simulink model "Virtual_Exhaust_Aftertreatment_Controller_PRT"  (R2016b)
settings: Solver=FixedStepAuto  StartTime=0.0  StopTime=inf  FixedStep=VirtExhATCtrlr.tiSimnTiStep_C  RelTol=1e-3  SampleTimeConstraint=STIndependent  EnableMultiTasking=on
undefined symbols (not defined in the file or in its folder): CAL, SOUIT, T3LIMCL_COEOM_MSK_SY, T3LimCL_stMskEOM1_C, T3LimCL_stMskEOM2_C, T3LimCL_stMskEOM3_C, VirtExhATCtrlr_numHrznSize_CA
libraries: simulink x4
(part 4 of 5)

== system Virtual_Exhaust_Aftertreatment_Controller_PRT/UCatCtrl/Urea_Dosing_Control/Load Governor/Saturation Dynamic ==
  up : Inport
  u : Inport  Port=2
  lo : Inport  Port=3
  Data Type Duplicate : DataTypeDuplicate  DisableCoverage=on
  Data Type Propagation : S-Function  FunctionName=sfix_dtprop  Parameters=14,PropDataTypeMode,(getdatatypespecs(PropDataType,PropScaling,DblOver,0, 0, PropDataTypeMode, PropScalingMode)),IfRefDouble,IfRefSingle,IsSigned,NumBitsBase,NumBitsMult,NumBitsAdd,(sort(reshape(round(NumBitsAllowFinal), prod(size(NumBitsAllowFinal)),1))),PropScalingMode,ValuesUsedBestPrec,SlopeBase,SlopeMult,SlopeAdd,BiasBase,BiasMult,BiasAdd,DblOver  SFunctionDeploymentMode=off  EnableBusSupport=off  mask(Data Type Propagation){PropDataTypeMode=Inherit via propagation rule, PropDataType=fixdt(1, 16), IfRefDouble=double, IfRefSingle=single, IsSigned=IsSigned1, NumBitsBase=NumBits1, NumBitsMult=1, NumBitsAdd=0, NumBitsAllowFinal=1:128, PropScalingMode=Inherit via propagation rule, PropScaling=2^-10, ValuesUsedBestPrec=[5 -7], SlopeBase=Slope1, SlopeMult=1, SlopeAdd=0, BiasBase=Bias1, BiasMult=1, BiasAdd=0}
      mask prompts: PropDataTypeMode "Simulink:masks:x1PropagatedDataType_MP"; PropDataType "Simulink:masks:x11PropagatedDataTypeegFixdt116Fixdtsingle_MP"; IfRefDouble "Simulink:masks:x11IfAnyReferenceInputIsDoubleOutputIs_MP"; IfRefSingle "Simulink:masks:x12IfAnyReferenceInputIsSingleOutputIs_MP"; IsSigned "Simulink:masks:x13IsSigned_MP"; NumBitsBase "Simulink:masks:x141NumberofBitsBase_MP"; NumBitsMult "Simulink:masks:x142NumberofBitsMultiplicativeAdjustment_MP"; NumBitsAdd "Simulink:masks:x143NumberofBitsAdditiveAdjustment_MP"; NumBitsAllowFinal "Simulink:masks:x144NumberofBitsAllowableFinalValues_MP"; PropScalingMode "Simulink:masks:x2PropagatedScaling_MP"; PropScaling "Simulink:masks:x21PropagatedScalingSlopeEg29OrSlopeBiasEg1253_MP"; ValuesUsedBestPrec "Simulink:masks:x21ValuesUsedToDetermineBestPrecisionScaling_MP"; SlopeBase "Simulink:masks:x211SlopeBase_MP"; SlopeMult "Simulink:masks:x212SlopeMultiplicativeAdjustment_MP"; SlopeAdd "Simulink:masks:x213SlopeAdditiveAdjustment_MP"; BiasBase "Simulink:masks:x221BiasBase_MP"; BiasMult "Simulink:masks:x222BiasMultiplicativeAdjustment_MP"; BiasAdd "Simulink:masks:x223BiasAdditiveAdjustment_MP"
      mask help: Simulink:masks:DataTypePropagation_MD
      mask init:
      | DblOver = 0;
      mask TypeOptions PropDataTypeMode: Simulink:masks:SpecifyViaDialog | Simulink:masks:InheritViaPropagationRule
      mask Callback PropDataTypeMode: fixptdialog(gcbh)
      mask Callback PropDataType: fixptdialog(gcbh)
      mask TypeOptions IfRefDouble: Simulink:masks:double | Simulink:masks:single
      mask TypeOptions IfRefSingle: Simulink:masks:double | Simulink:masks:single
      mask TypeOptions IsSigned: Simulink:masks:IsSigned1 | Simulink:masks:IsSigned2 | Simulink:masks:IsSigned1OrIsSigned2 | Simulink:masks:TRUE | Simulink:masks:FALSE
      mask TypeOptions NumBitsBase: NumBits1 | NumBits2 | max([NumBits1 NumBits2]) | min([NumBits1 NumBits2]) | NumBits1+NumBits2
      mask TypeOptions PropScalingMode: Simulink:masks:SpecifyViaDialog | Simulink:masks:InheritViaPropagationRule | Simulink:masks:ObtainViaBestPrecision
      mask Callback PropScalingMode: fixptdialog(gcbh)
      mask TypeOptions SlopeBase: Slope1 | Slope2 | max([Slope1 Slope2]) | min([Slope1 Slope2]) | Slope1*Slope2 | Slope1/Slope2 | PosRange1 | PosRange2 | max([PosRange1 PosRange2]) | min([PosRange1 PosRange2]) | PosRange1*PosRange2 | PosRange1/PosRange2
      mask TypeOptions BiasBase: Bias1 | Bias2 | max([Bias1 Bias2]) | min([Bias1 Bias2]) | Bias1*Bias2 | Bias1/Bias2 | Bias1+Bias2 | Bias1-Bias2
      mask Display:
      | port_label('Input',1,'Ref1');
      | port_label('Input',2,'Ref2');
      | port_label('Input',3,'Prop');
  LowerRelop1 : RelationalOperator  DisableCoverage=on  Operator=>  OutDataTypeStr=boolean  RndMeth=Nearest
  Switch : Switch  Criteria=u2 ~= 0  OutDataTypeStr=Inherit: Inherit via back propagation  ZeroCross=off
  Switch2 : Switch  Criteria=u2 ~= 0  OutMin=OutMin  OutMax=OutMax  OutDataTypeStr=Inherit: Inherit via back propagation  ZeroCross=off
  UpperRelop : RelationalOperator  DisableCoverage=on  Operator=<  OutDataTypeStr=boolean  RndMeth=Nearest
  y : Outport  OutMin=OutMin  OutMax=OutMax
  wires:
  up/1 -> Switch2/1, LowerRelop1/2
  u/1 -> Data Type Propagation/2, Data Type Propagation/1, LowerRelop1/1, Switch/3, UpperRelop/1
  lo/1 -> Switch/1, UpperRelop/2
  Switch/1 -> Data Type Duplicate/2, Switch2/3, Data Type Propagation/3
  Switch2/1 -> Data Type Duplicate/1, y/1
  LowerRelop1/1 -> Switch2/2
  UpperRelop/1 -> Switch/2

== system Virtual_Exhaust_Aftertreatment_Controller_PRT/UCatCtrl/SCR_Prediction/Main/Aging Prediction/estAging ==
  ATS_tAvrg : Inport
  ATS_GlbDa_ITotDst : Inport  Port=2
  Constant1 : Constant  Value=CAL.SCALAR.SCRMod_facSCRAgeSca_C  OutDataTypeStr=Inherit: Inherit via back propagation  SampleTime=-1
  Constant10 : Constant  Value=CAL.SCALAR.SCRMod_facSCRAgeTempSca_C  OutDataTypeStr=Inherit: Inherit via back propagation  SampleTime=-1
  Constant2 : Constant  Value=32767  SampleTime=-1
  MinMax : MinMax  Inputs=2
  MinMax1 : MinMax  Inputs=2
  Product : Product
  Product1 : Product
  SCRMod_facEffSCRAge_MAP : Lookup_n-D  BreakpointsForDimension1=CAL.TABLE.SCRMod_facEffSCRAge_MAP.Y  BreakpointsForDimension2=CAL.TABLE.SCRMod_facEffSCRAge_MAP.X  Table=CAL.TABLE.SCRMod_facEffSCRAge_MAP.Z  ExtrapMethod=Clip  UseLastTableValue=on  RndMeth=Simplest  InputSameDT=on
  SCRMod_facTempSCRAge_CUR : Lookup_n-D  NumberOfTableDimensions=1  BreakpointsForDimension1=CAL.TABLE.SCRMod_facTempSCRAge_MAP.X  BreakpointsForDimension2=CAL.TABLE.SCRMod_facEffSCRAge_MAP.X  Table=CAL.TABLE.SCRMod_facTempSCRAge_MAP.Y  ExtrapMethod=Clip  UseLastTableValue=on  RndMeth=Simplest  InputSameDT=on
  ATS_facEstEfcUCatAge : Outport
  wires:
  ATS_tAvrg/1 -> SCRMod_facTempSCRAge_CUR/1
  SCRMod_facTempSCRAge_CUR/1 -> Product1/1
  Constant10/1 -> Product1/2
  Product1/1 -> MinMax/1
  Constant2/1 -> MinMax1/1, MinMax/2
  Product/1 -> MinMax1/2
  MinMax/1 -> SCRMod_facEffSCRAge_MAP/1
  MinMax1/1 -> SCRMod_facEffSCRAge_MAP/2
  SCRMod_facEffSCRAge_MAP/1 -> ATS_facEstEfcUCatAge/1
  ATS_GlbDa_ITotDst/1 -> Product/1
  Constant1/1 -> Product/2

== system Virtual_Exhaust_Aftertreatment_Controller_PRT/UCatCtrl/SCR_Prediction/Main/UCat Efficiency Prediction/SubSystem_10 ==
  In1 : Inport
  In2 : Inport  Port=2
  In3 : Inport  Port=3
  In4 : Inport  Port=4
  Interpolation Using Prelookup : Interpolation_n-D  Table=table  ExtrapMethod=Clip  ValidIndexMayReachLast=on
  Out1 : Outport
  wires:
  Interpolation Using Prelookup/1 -> Out1/1
  In1/1 -> Interpolation Using Prelookup/1
  In2/1 -> Interpolation Using Prelookup/2
  In3/1 -> Interpolation Using Prelookup/3
  In4/1 -> Interpolation Using Prelookup/4

== system Virtual_Exhaust_Aftertreatment_Controller_PRT/UCatCtrl/SCR_Prediction/Main/UCat Efficiency Prediction/SubSystem_11 ==
  In1 : Inport
  In2 : Inport  Port=2
  In3 : Inport  Port=3
  In4 : Inport  Port=4
  Interpolation Using Prelookup : Interpolation_n-D  Table=table  ExtrapMethod=Clip  ValidIndexMayReachLast=on
  Out1 : Outport
  wires:
  In4/1 -> Interpolation Using Prelookup/4
  In3/1 -> Interpolation Using Prelookup/3
  In2/1 -> Interpolation Using Prelookup/2
  In1/1 -> Interpolation Using Prelookup/1
  Interpolation Using Prelookup/1 -> Out1/1

== system Virtual_Exhaust_Aftertreatment_Controller_PRT/UCatCtrl/SCR_Prediction/Main/UCat Efficiency Prediction/SubSystem_12 ==
  In1 : Inport
  In2 : Inport  Port=2
  In3 : Inport  Port=3
  In4 : Inport  Port=4
  Interpolation Using Prelookup : Interpolation_n-D  Table=table  ExtrapMethod=Clip  ValidIndexMayReachLast=on
  Out1 : Outport
  wires:
  In4/1 -> Interpolation Using Prelookup/4
  In3/1 -> Interpolation Using Prelookup/3
  In2/1 -> Interpolation Using Prelookup/2
  In1/1 -> Interpolation Using Prelookup/1
  Interpolation Using Prelookup/1 -> Out1/1

== system Virtual_Exhaust_Aftertreatment_Controller_PRT/UCatCtrl/SCR_Prediction/Main/UCat Efficiency Prediction/SubSystem_3 ==
  In1 : Inport
  In2 : Inport  Port=2
  In3 : Inport  Port=3
  In4 : Inport  Port=4
  Interpolation Using Prelookup : Interpolation_n-D  Table=table  ExtrapMethod=Clip  ValidIndexMayReachLast=on
  Out1 : Outport
  wires:
  Interpolation Using Prelookup/1 -> Out1/1
  In1/1 -> Interpolation Using Prelookup/1
  In2/1 -> Interpolation Using Prelookup/2
  In3/1 -> Interpolation Using Prelookup/3
  In4/1 -> Interpolation Using Prelookup/4

== system Virtual_Exhaust_Aftertreatment_Controller_PRT/UCatCtrl/SCR_Prediction/Main/UCat Efficiency Prediction/SubSystem_4 ==
  In1 : Inport
  In2 : Inport  Port=2
  In3 : Inport  Port=3
  In4 : Inport  Port=4
  Interpolation Using Prelookup : Interpolation_n-D  Table=table  ExtrapMethod=Clip  ValidIndexMayReachLast=on
  Out1 : Outport
  wires:
  In4/1 -> Interpolation Using Prelookup/4
  In3/1 -> Interpolation Using Prelookup/3
  In2/1 -> Interpolation Using Prelookup/2
  In1/1 -> Interpolation Using Prelookup/1
  Interpolation Using Prelookup/1 -> Out1/1

== system Virtual_Exhaust_Aftertreatment_Controller_PRT/UCatCtrl/SCR_Prediction/Main/UCat Efficiency Prediction/SubSystem_5 ==
  In1 : Inport
  In2 : Inport  Port=2
  In3 : Inport  Port=3
  In4 : Inport  Port=4
  Interpolation Using Prelookup : Interpolation_n-D  Table=table  ExtrapMethod=Clip  ValidIndexMayReachLast=on
  Out1 : Outport
  wires:
  Interpolation Using Prelookup/1 -> Out1/1
  In1/1 -> Interpolation Using Prelookup/1
  In2/1 -> Interpolation Using Prelookup/2
  In3/1 -> Interpolation Using Prelookup/3
  In4/1 -> Interpolation Using Prelookup/4

== system Virtual_Exhaust_Aftertreatment_Controller_PRT/UCatCtrl/SCR_Prediction/Main/UCat Efficiency Prediction/SubSystem_6 ==
  In1 : Inport
  In2 : Inport  Port=2
  In3 : Inport  Port=3
  In4 : Inport  Port=4
  Interpolation Using Prelookup : Interpolation_n-D  Table=table  ExtrapMethod=Clip  ValidIndexMayReachLast=on
  Out1 : Outport
  wires:
  In4/1 -> Interpolation Using Prelookup/4
  In3/1 -> Interpolation Using Prelookup/3
  In2/1 -> Interpolation Using Prelookup/2
  In1/1 -> Interpolation Using Prelookup/1
  Interpolation Using Prelookup/1 -> Out1/1

== system Virtual_Exhaust_Aftertreatment_Controller_PRT/UCatCtrl/SCR_Prediction/Main/UCat Efficiency Prediction/SubSystem_7 ==
  In1 : Inport
  In2 : Inport  Port=2
  In3 : Inport  Port=3
  In4 : Inport  Port=4
  Interpolation Using Prelookup : Interpolation_n-D  Table=table  ExtrapMethod=Clip  ValidIndexMayReachLast=on
  Out1 : Outport
  wires:
  Interpolation Using Prelookup/1 -> Out1/1
  In1/1 -> Interpolation Using Prelookup/1
  In2/1 -> Interpolation Using Prelookup/2
  In3/1 -> Interpolation Using Prelookup/3
  In4/1 -> Interpolation Using Prelookup/4

== system Virtual_Exhaust_Aftertreatment_Controller_PRT/UCatCtrl/SCR_Prediction/Main/UCat Efficiency Prediction/SubSystem_8 ==
  In1 : Inport
  In2 : Inport  Port=2
  In3 : Inport  Port=3
  In4 : Inport  Port=4
  Interpolation Using Prelookup : Interpolation_n-D  Table=table  ExtrapMethod=Clip  ValidIndexMayReachLast=on
  Out1 : Outport
  wires:
  Interpolation Using Prelookup/1 -> Out1/1
  In1/1 -> Interpolation Using Prelookup/1
  In2/1 -> Interpolation Using Prelookup/2
  In3/1 -> Interpolation Using Prelookup/3
  In4/1 -> Interpolation Using Prelookup/4

== system Virtual_Exhaust_Aftertreatment_Controller_PRT/UCatCtrl/SCR_Prediction/Main/UCat Efficiency Prediction/SubSystem_9 ==
  In1 : Inport
  In2 : Inport  Port=2
  In3 : Inport  Port=3
  In4 : Inport  Port=4
  Interpolation Using Prelookup : Interpolation_n-D  Table=table  ExtrapMethod=Clip  ValidIndexMayReachLast=on
  Out1 : Outport
  wires:
  In4/1 -> Interpolation Using Prelookup/4
  In3/1 -> Interpolation Using Prelookup/3
  In2/1 -> Interpolation Using Prelookup/2
  In1/1 -> Interpolation Using Prelookup/1
  Interpolation Using Prelookup/1 -> Out1/1

== system Virtual_Exhaust_Aftertreatment_Controller_PRT/UCatCtrl/SCR_Prediction/Main/UCat NH3 Load Prediction/Discrete Integrator ==
  X : Inport
  Ki : Inport  Port=2
  Reset : Inport  Port=3
  Y0_YReset : Inport  Port=4
  Min : Inport  Port=5
  Max : Inport  Port=6
  dT : Inport  Port=7
  Add1 : Sum
  Add2 : Sum
  AntiWindUp : Subsystem
  Constant2 : Constant  Value=0  SampleTime=-1
  Constant3 : Constant  Value=0  SampleTime=-1
  Kp = 0 : Constant  SampleTime=-1
  Product1 : Product  RndMeth=Zero
  Product2 : Product  RndMeth=Zero
  Product3 : Product  RndMeth=Zero
  Saturation : Subsystem
  Switch1 : Switch  Criteria=u2 ~= 0
  Switch2 : Switch  Criteria=u2 ~= 0
  Switch3 : Switch  Criteria=u2 ~= 0
  Unit Delay External IC : Subsystem  mask(Unit Delay External Initial Condition){tsamp=-1}
      mask prompts: tsamp "Simulink:masks:SampleTime_MP"
      mask help: Simulink:masks:UnitDelayExternalInitialCondition_MD
      mask Display: dpoly(1,[1 0],'z')
  Unit Delay External IC1 : Subsystem  mask(Unit Delay External Initial Condition){tsamp=-1}
      mask prompts: tsamp "Simulink:masks:SampleTime_MP"
      mask help: Simulink:masks:UnitDelayExternalInitialCondition_MD
      mask Display: dpoly(1,[1 0],'z')
  Y : Outport
  wires:
  Unit Delay External IC1/1(y) -> Y/1
  X/1 -> Product2/1, Product1/1
  Kp = 0/1 -> Product1/2
  Ki/1 -> Product2/2
  Product2/1 -> Product3/1
  dT/1 -> Product3/2
  Product3/1 -> AntiWindUp/1(PreInteg), Switch1/3
  Unit Delay External IC/1(y) -> Add1/2
  Max/1 -> Saturation/1(Max)
  Min/1 -> Saturation/3(Min)
  Switch1/1 -> Add1/1
  Constant2/1 -> Switch1/1
  AntiWindUp/1(Clamp) -> Switch1/2
  Saturation/2(Sat) -> AntiWindUp/2(Sat)
  Add1/1 -> Switch2/3
  Reset/1 -> Switch2/2, Switch3/2
  Y0_YReset/1 -> Switch2/1, Unit Delay External IC/2(IC), Unit Delay External IC1/2(IC)
  Product1/1 -> Switch3/3
  Constant3/1 -> Switch3/1
  Saturation/1(Y) -> Unit Delay External IC/1(u), Add2/2
  Switch3/1 -> Add2/1
  Add2/1 -> Unit Delay External IC1/1(u)
  Switch2/1 -> Saturation/2(X)

== system Virtual_Exhaust_Aftertreatment_Controller_PRT/UCatCtrl/SCR_Prediction/Main/UCat NH3 Load Prediction/GOTO_ATS_mflNH3OxiUCatUs_mgps ==
  InXX : Inport
  GainXX : Subsystem
  tag scope: ATS_mflNH3OxiUCatUs_mgps=global
  wires:
  GainXX/1(Out) -> [ATS_mflNH3OxiUCatUs_mgps]  "ATS_mflNH3OxiUCatUs_mgps"
  InXX/1 -> GainXX/1(In)

== system Virtual_Exhaust_Aftertreatment_Controller_PRT/UCatCtrl/SCR_Prediction/Main/UCat NH3 Load Prediction/NH3 Oxidation ==
  ATS_tEstUCatAvrg : Inport
  ATS_mflEG : Inport  Port=2
  ATS_mflNH3MetAdapDes_mgps : Inport  Port=3
  ATS_facEffUCatAge : Inport  Port=4
  ATS_mEstNH3LdUCat : Inport  Port=5
  NH3 Oxidation : Subsystem
  mg/s to ppm : Subsystem
  ATS_mflNH3OxiUCatUs_mgps : Outport
  wires:
  ATS_tEstUCatAvrg/1 -> NH3 Oxidation/2(ATS_tEstUCatAvrg)
  ATS_mEstNH3LdUCat/1 -> NH3 Oxidation/1(ATS_mEstNH3LdUCat)
  ATS_mflEG/1 -> NH3 Oxidation/4("ATS_mflEG "), mg/s to ppm/2(ATS_mflEG)
  ATS_mflNH3MetAdapDes_mgps/1 -> mg/s to ppm/1(ATS_mflNH3MetAdapDes_mgps)
  mg/s to ppm/1(ATS_rNH3Curr_ppm) -> NH3 Oxidation/3(ATS_rNH3Curr_ppm)
  ATS_facEffUCatAge/1 -> NH3 Oxidation/5(ATS_facEffUCatAge)
  NH3 Oxidation/1(ATS_mflNH3OxiUCatUs_mgps) -> ATS_mflNH3OxiUCatUs_mgps/1

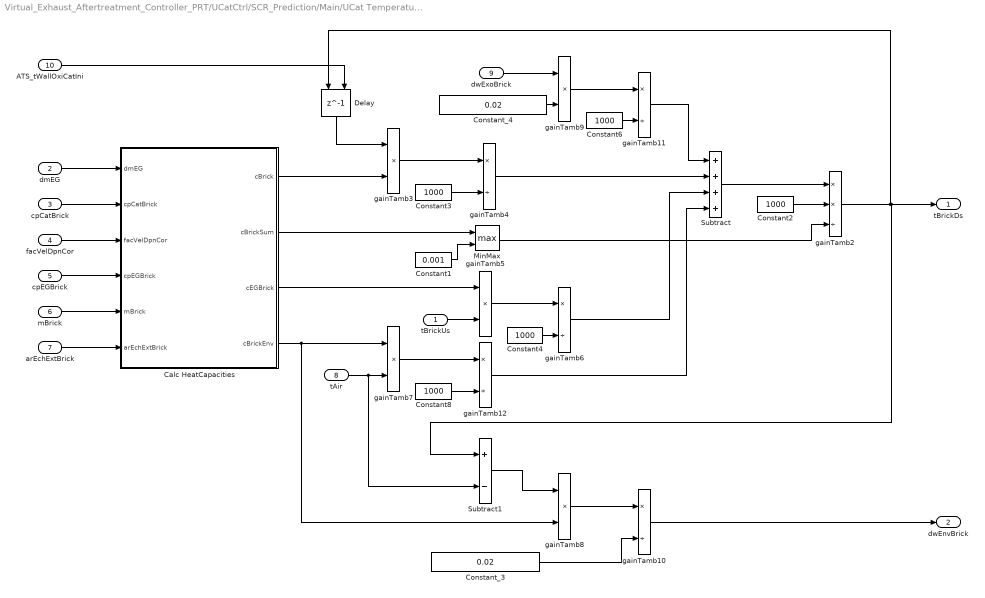
== system Virtual_Exhaust_Aftertreatment_Controller_PRT/UCatCtrl/SCR_Prediction/Main/UCat Temperature Prediction/DOC Temperature Estimation 1 ==
  tBrickUs : Inport
  dmEG : Inport  Port=2
  cpCatBrick : Inport  Port=3
  facVelDpnCor : Inport  Port=4
  cpEGBrick : Inport  Port=5
  mBrick : Inport  Port=6
  arEchExtBrick : Inport  Port=7
  tAir : Inport  Port=8
  dwExoBrick : Inport  Port=9
  ATS_tWallOxiCatIni : Inport  Port=10
  Calc HeatCapacities : Subsystem  TreatAsAtomicUnit=on
  Constant1 : Constant  Value=0.001  SampleTime=-1
  Constant{2..4,6,8} (5 alike) : Constant  Value=1000  SampleTime=-1
  Constant_3 : Constant  Value=0.02  SampleTime=-1
  Constant_4 : Constant  Value=0.02  SampleTime=-1
  Delay : Delay  DelayLength=1  InitialConditionSource=Input port  InitialCondition=0
      settings: InputPortMap=u0,p4
  MinMax : MinMax  Function=max  Inputs=2
  Subtract : Sum  Inputs=++++
  Subtract1 : Sum  Inputs=+-
  gainTamb{4,6,10..12} (5 alike) : Product  Inputs=*/  SaturateOnIntegerOverflow=on  InputSameDT=on  OutDataTypeStr=Inherit: Same as first input
  gainTamb2 : Product  Inputs=**/  SaturateOnIntegerOverflow=on  InputSameDT=on  OutDataTypeStr=Inherit: Same as first input
  gainTamb{3,5,7..9} (5 alike) : Product  Inputs=**  SaturateOnIntegerOverflow=on  InputSameDT=on  OutDataTypeStr=Inherit: Same as first input
  tBrickDs : Outport
  dwEnvBrick : Outport  Port=2
  wires:
  dmEG/1 -> Calc HeatCapacities/1(dmEG)
  cpCatBrick/1 -> Calc HeatCapacities/2(cpCatBrick)
  facVelDpnCor/1 -> Calc HeatCapacities/3(facVelDpnCor)
  cpEGBrick/1 -> Calc HeatCapacities/4(cpEGBrick)
  mBrick/1 -> Calc HeatCapacities/5(mBrick)
  arEchExtBrick/1 -> Calc HeatCapacities/6(arEchExtBrick)
  Calc HeatCapacities/2(cBrickSum) -> MinMax/1
  Constant1/1 -> MinMax/2
  Subtract/1 -> gainTamb2/1
  Constant2/1 -> gainTamb2/2
  MinMax/1 -> gainTamb2/3
  gainTamb2/1 -> Subtract1/1, tBrickDs/1, Delay/1
  Calc HeatCapacities/1(cBrick) -> gainTamb3/2
  gainTamb3/1 -> gainTamb4/1
  Constant3/1 -> gainTamb4/2
  gainTamb4/1 -> Subtract/2
  Calc HeatCapacities/3(cEGBrick) -> gainTamb5/1
  tBrickUs/1 -> gainTamb5/2
  gainTamb5/1 -> gainTamb6/1
  Constant4/1 -> gainTamb6/2
  Calc HeatCapacities/4(cBrickEnv) -> gainTamb8/2, gainTamb7/1
  tAir/1 -> gainTamb7/2, Subtract1/2
  Subtract1/1 -> gainTamb8/1
  gainTamb8/1 -> gainTamb10/1
  Constant_3/1 -> gainTamb10/2
  gainTamb10/1 -> dwEnvBrick/1
  gainTamb6/1 -> Subtract/3
  dwExoBrick/1 -> gainTamb9/1
  gainTamb9/1 -> gainTamb11/1
  Constant6/1 -> gainTamb11/2
  Constant_4/1 -> gainTamb9/2
  gainTamb11/1 -> Subtract/1
  gainTamb7/1 -> gainTamb12/1
  Constant8/1 -> gainTamb12/2
  gainTamb12/1 -> Subtract/4
  Delay/1 -> gainTamb3/1
  ATS_tWallOxiCatIni/1 -> Delay/2

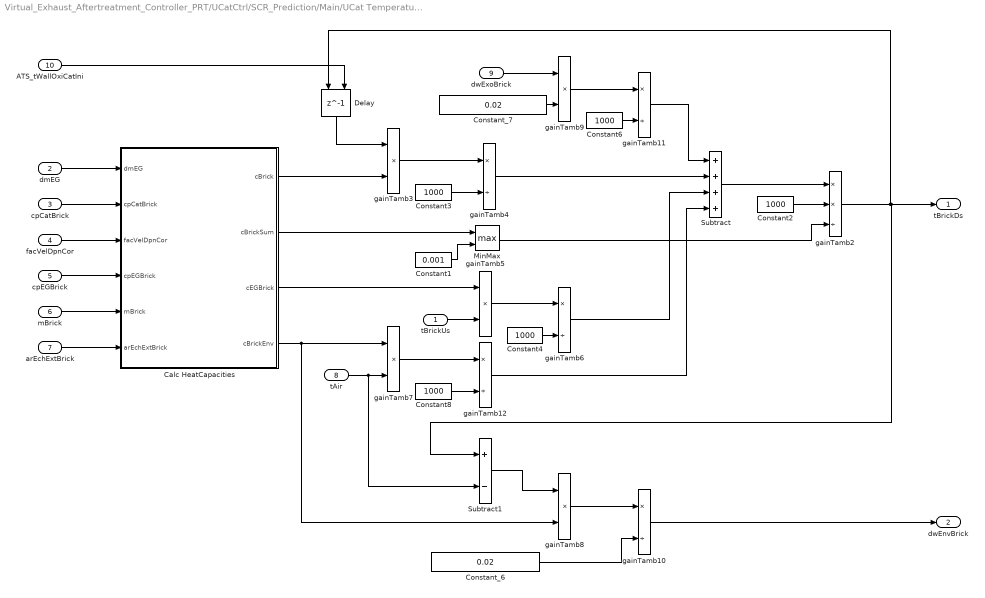
== system Virtual_Exhaust_Aftertreatment_Controller_PRT/UCatCtrl/SCR_Prediction/Main/UCat Temperature Prediction/DOC Temperature Estimation 2 ==
  tBrickUs : Inport
  dmEG : Inport  Port=2
  cpCatBrick : Inport  Port=3
  facVelDpnCor : Inport  Port=4
  cpEGBrick : Inport  Port=5
  mBrick : Inport  Port=6
  arEchExtBrick : Inport  Port=7
  tAir : Inport  Port=8
  dwExoBrick : Inport  Port=9
  ATS_tWallOxiCatIni : Inport  Port=10
  Calc HeatCapacities : Subsystem  TreatAsAtomicUnit=on
  Constant1 : Constant  Value=0.001  SampleTime=-1
  Constant{2..4,6,8} (5 alike) : Constant  Value=1000  SampleTime=-1
  Constant_6 : Constant  Value=0.02  SampleTime=-1
  Constant_7 : Constant  Value=0.02  SampleTime=-1
  Delay : Delay  DelayLength=1  InitialConditionSource=Input port  InitialCondition=0
      settings: InputPortMap=u0,p4
  MinMax : MinMax  Function=max  Inputs=2
  Subtract : Sum  Inputs=++++
  Subtract1 : Sum  Inputs=+-
  gainTamb{4,6,10..12} (5 alike) : Product  Inputs=*/  SaturateOnIntegerOverflow=on  InputSameDT=on  OutDataTypeStr=Inherit: Same as first input
  gainTamb2 : Product  Inputs=**/  SaturateOnIntegerOverflow=on  InputSameDT=on  OutDataTypeStr=Inherit: Same as first input
  gainTamb{3,5,7..9} (5 alike) : Product  Inputs=**  SaturateOnIntegerOverflow=on  InputSameDT=on  OutDataTypeStr=Inherit: Same as first input
  tBrickDs : Outport
  dwEnvBrick : Outport  Port=2
  wires:
  dmEG/1 -> Calc HeatCapacities/1(dmEG)
  cpCatBrick/1 -> Calc HeatCapacities/2(cpCatBrick)
  facVelDpnCor/1 -> Calc HeatCapacities/3(facVelDpnCor)
  cpEGBrick/1 -> Calc HeatCapacities/4(cpEGBrick)
  mBrick/1 -> Calc HeatCapacities/5(mBrick)
  arEchExtBrick/1 -> Calc HeatCapacities/6(arEchExtBrick)
  Calc HeatCapacities/2(cBrickSum) -> MinMax/1
  Constant1/1 -> MinMax/2
  Subtract/1 -> gainTamb2/1
  Constant2/1 -> gainTamb2/2
  MinMax/1 -> gainTamb2/3
  gainTamb2/1 -> Subtract1/1, tBrickDs/1, Delay/1
  Calc HeatCapacities/1(cBrick) -> gainTamb3/2
  gainTamb3/1 -> gainTamb4/1
  Constant3/1 -> gainTamb4/2
  gainTamb4/1 -> Subtract/2
  Calc HeatCapacities/3(cEGBrick) -> gainTamb5/1
  tBrickUs/1 -> gainTamb5/2
  gainTamb5/1 -> gainTamb6/1
  Constant4/1 -> gainTamb6/2
  Calc HeatCapacities/4(cBrickEnv) -> gainTamb8/2, gainTamb7/1
  tAir/1 -> gainTamb7/2, Subtract1/2
  Subtract1/1 -> gainTamb8/1
  gainTamb8/1 -> gainTamb10/1
  Constant_6/1 -> gainTamb10/2
  gainTamb10/1 -> dwEnvBrick/1
  gainTamb6/1 -> Subtract/3
  dwExoBrick/1 -> gainTamb9/1
  gainTamb9/1 -> gainTamb11/1
  Constant6/1 -> gainTamb11/2
  Constant_7/1 -> gainTamb9/2
  gainTamb11/1 -> Subtract/1
  gainTamb7/1 -> gainTamb12/1
  Constant8/1 -> gainTamb12/2
  gainTamb12/1 -> Subtract/4
  Delay/1 -> gainTamb3/1
  ATS_tWallOxiCatIni/1 -> Delay/2

== system Virtual_Exhaust_Aftertreatment_Controller_PRT/UCatCtrl/SCR_Prediction/Main/UCat Temperature Prediction/DOC Temperature Estimation 3 ==
  tBrickUs : Inport
  dmEG : Inport  Port=2
  cpCatBrick : Inport  Port=3
  facVelDpnCor : Inport  Port=4
  cpEGBrick : Inport  Port=5
  mBrick : Inport  Port=6
  arEchExtBrick : Inport  Port=7
  tAir : Inport  Port=8
  dwExoBrick : Inport  Port=9
  ATS_tWallOxiCatIni : Inport  Port=10
  Calc HeatCapacities : Subsystem  TreatAsAtomicUnit=on
  Constant1 : Constant  Value=0.001  SampleTime=-1
  Constant{2..4,6,8} (5 alike) : Constant  Value=1000  SampleTime=-1
  Constant_10 : Constant  Value=0.02  SampleTime=-1
  Constant_9 : Constant  Value=0.02  SampleTime=-1
  Delay : Delay  DelayLength=1  InitialConditionSource=Input port  InitialCondition=0
      settings: InputPortMap=u0,p4
  MinMax : MinMax  Function=max  Inputs=2
  Subtract : Sum  Inputs=++++
  Subtract1 : Sum  Inputs=+-
  gainTamb{4,6,10..12} (5 alike) : Product  Inputs=*/  SaturateOnIntegerOverflow=on  InputSameDT=on  OutDataTypeStr=Inherit: Same as first input
  gainTamb2 : Product  Inputs=**/  SaturateOnIntegerOverflow=on  InputSameDT=on  OutDataTypeStr=Inherit: Same as first input
  gainTamb{3,5,7..9} (5 alike) : Product  Inputs=**  SaturateOnIntegerOverflow=on  InputSameDT=on  OutDataTypeStr=Inherit: Same as first input
  tBrickDs : Outport
  dwEnvBrick : Outport  Port=2
  wires:
  dmEG/1 -> Calc HeatCapacities/1(dmEG)
  cpCatBrick/1 -> Calc HeatCapacities/2(cpCatBrick)
  facVelDpnCor/1 -> Calc HeatCapacities/3(facVelDpnCor)
  cpEGBrick/1 -> Calc HeatCapacities/4(cpEGBrick)
  mBrick/1 -> Calc HeatCapacities/5(mBrick)
  arEchExtBrick/1 -> Calc HeatCapacities/6(arEchExtBrick)
  Calc HeatCapacities/2(cBrickSum) -> MinMax/1
  Constant1/1 -> MinMax/2
  Subtract/1 -> gainTamb2/1
  Constant2/1 -> gainTamb2/2
  MinMax/1 -> gainTamb2/3
  gainTamb2/1 -> Subtract1/1, tBrickDs/1, Delay/1
  Calc HeatCapacities/1(cBrick) -> gainTamb3/2
  gainTamb3/1 -> gainTamb4/1
  Constant3/1 -> gainTamb4/2
  gainTamb4/1 -> Subtract/2
  Calc HeatCapacities/3(cEGBrick) -> gainTamb5/1
  tBrickUs/1 -> gainTamb5/2
  gainTamb5/1 -> gainTamb6/1
  Constant4/1 -> gainTamb6/2
  Calc HeatCapacities/4(cBrickEnv) -> gainTamb8/2, gainTamb7/1
  tAir/1 -> gainTamb7/2, Subtract1/2
  Subtract1/1 -> gainTamb8/1
  gainTamb8/1 -> gainTamb10/1
  Constant_9/1 -> gainTamb10/2
  gainTamb10/1 -> dwEnvBrick/1
  gainTamb6/1 -> Subtract/3
  dwExoBrick/1 -> gainTamb9/1
  gainTamb9/1 -> gainTamb11/1
  Constant6/1 -> gainTamb11/2
  Constant_10/1 -> gainTamb9/2
  gainTamb11/1 -> Subtract/1
  gainTamb7/1 -> gainTamb12/1
  Constant8/1 -> gainTamb12/2
  gainTamb12/1 -> Subtract/4
  Delay/1 -> gainTamb3/1
  ATS_tWallOxiCatIni/1 -> Delay/2

== system Virtual_Exhaust_Aftertreatment_Controller_PRT/UCatCtrl/SCR_Prediction/Main/UCat Temperature Prediction/DOC Temperature Estimation 4 ==
  tBrickUs : Inport
  dmEG : Inport  Port=2
  cpCatBrick : Inport  Port=3
  facVelDpnCor : Inport  Port=4
  cpEGBrick : Inport  Port=5
  mBrick : Inport  Port=6
  arEchExtBrick : Inport  Port=7
  tAir : Inport  Port=8
  dwExoBrick : Inport  Port=9
  ATS_tWallOxiCatIni : Inport  Port=10
  Calc HeatCapacities : Subsystem  TreatAsAtomicUnit=on
  Constant1 : Constant  Value=0.001  SampleTime=-1
  Constant{2..4,6,8} (5 alike) : Constant  Value=1000  SampleTime=-1
  Constant_12 : Constant  Value=0.02  SampleTime=-1
  Constant_13 : Constant  Value=0.02  SampleTime=-1
  Delay : Delay  DelayLength=1  InitialConditionSource=Input port  InitialCondition=0
      settings: InputPortMap=u0,p4
  MinMax : MinMax  Function=max  Inputs=2
  Subtract : Sum  Inputs=++++
  Subtract1 : Sum  Inputs=+-
  gainTamb{4,6,10..12} (5 alike) : Product  Inputs=*/  SaturateOnIntegerOverflow=on  InputSameDT=on  OutDataTypeStr=Inherit: Same as first input
  gainTamb2 : Product  Inputs=**/  SaturateOnIntegerOverflow=on  InputSameDT=on  OutDataTypeStr=Inherit: Same as first input
  gainTamb{3,5,7..9} (5 alike) : Product  Inputs=**  SaturateOnIntegerOverflow=on  InputSameDT=on  OutDataTypeStr=Inherit: Same as first input
  tBrickDs : Outport
  dwEnvBrick : Outport  Port=2
  wires:
  dmEG/1 -> Calc HeatCapacities/1(dmEG)
  cpCatBrick/1 -> Calc HeatCapacities/2(cpCatBrick)
  facVelDpnCor/1 -> Calc HeatCapacities/3(facVelDpnCor)
  cpEGBrick/1 -> Calc HeatCapacities/4(cpEGBrick)
  mBrick/1 -> Calc HeatCapacities/5(mBrick)
  arEchExtBrick/1 -> Calc HeatCapacities/6(arEchExtBrick)
  Calc HeatCapacities/2(cBrickSum) -> MinMax/1
  Constant1/1 -> MinMax/2
  Subtract/1 -> gainTamb2/1
  Constant2/1 -> gainTamb2/2
  MinMax/1 -> gainTamb2/3
  gainTamb2/1 -> Subtract1/1, tBrickDs/1, Delay/1
  Calc HeatCapacities/1(cBrick) -> gainTamb3/2
  gainTamb3/1 -> gainTamb4/1
  Constant3/1 -> gainTamb4/2
  gainTamb4/1 -> Subtract/2
  Calc HeatCapacities/3(cEGBrick) -> gainTamb5/1
  tBrickUs/1 -> gainTamb5/2
  gainTamb5/1 -> gainTamb6/1
  Constant4/1 -> gainTamb6/2
  Calc HeatCapacities/4(cBrickEnv) -> gainTamb8/2, gainTamb7/1
  tAir/1 -> gainTamb7/2, Subtract1/2
  Subtract1/1 -> gainTamb8/1
  gainTamb8/1 -> gainTamb10/1
  Constant_12/1 -> gainTamb10/2
  gainTamb10/1 -> dwEnvBrick/1
  gainTamb6/1 -> Subtract/3
  dwExoBrick/1 -> gainTamb9/1
  gainTamb9/1 -> gainTamb11/1
  Constant6/1 -> gainTamb11/2
  Constant_13/1 -> gainTamb9/2
  gainTamb11/1 -> Subtract/1
  gainTamb7/1 -> gainTamb12/1
  Constant8/1 -> gainTamb12/2
  gainTamb12/1 -> Subtract/4
  Delay/1 -> gainTamb3/1
  ATS_tWallOxiCatIni/1 -> Delay/2

== system Virtual_Exhaust_Aftertreatment_Controller_PRT/UCatCtrl/SCR_Prediction/Main/UCat Temperature Prediction/Gas and Catalyst Properties1 ==
  tBrickUs : Inport
  tBrickDs : Inport  Port=2
  Lookup_2 : Lookup  InputValues=[-0.0400000000000091;49.96;99.96;199.96;299.96;399.96;499.96;599.96;699.96;799.96]  Table=[1;1.0375;1.075;1.15;1.2;1.25;1.3;1.35;1.4;1.4]  LookUpMeth=Interpolation-Use End Values
  Lookup_3 : Lookup  InputValues=[-100.04;-0.0400000000000091;99.96;199.96;299.96;399.96;499.96;599.96;699.96;799.96]  Table=[1;1.019;1.07;1.14;1.195;1.217;1.225;1.234;1.243;1.27]  LookUpMeth=Interpolation-Use End Values
  cpCatBrick : Outport
  cpEGBrick : Outport  Port=2
  wires:
  tBrickUs/1 -> Lookup_3/1
  Lookup_3/1 -> cpEGBrick/1
  Lookup_2/1 -> cpCatBrick/1
  tBrickDs/1 -> Lookup_2/1

== system Virtual_Exhaust_Aftertreatment_Controller_PRT/UCatCtrl/SCR_Prediction/Main/UCat Temperature Prediction/Gas and Catalyst Properties2 ==
  tBrickUs : Inport
  tBrickDs : Inport  Port=2
  Lookup_4 : Lookup  InputValues=[-0.0400000000000091;49.96;99.96;199.96;299.96;399.96;499.96;599.96;699.96;799.96]  Table=[1;1.0375;1.075;1.15;1.2;1.25;1.3;1.35;1.4;1.4]  LookUpMeth=Interpolation-Use End Values
  Lookup_5 : Lookup  InputValues=[-100.04;-0.0400000000000091;99.96;199.96;299.96;399.96;499.96;599.96;699.96;799.96]  Table=[1;1.019;1.07;1.14;1.195;1.217;1.225;1.234;1.243;1.27]  LookUpMeth=Interpolation-Use End Values
  cpCatBrick : Outport
  cpEGBrick : Outport  Port=2
  wires:
  tBrickUs/1 -> Lookup_5/1
  Lookup_5/1 -> cpEGBrick/1
  Lookup_4/1 -> cpCatBrick/1
  tBrickDs/1 -> Lookup_4/1

== system Virtual_Exhaust_Aftertreatment_Controller_PRT/UCatCtrl/SCR_Prediction/Main/UCat Temperature Prediction/Gas and Catalyst Properties3 ==
  tBrickUs : Inport
  tBrickDs : Inport  Port=2
  Lookup_6 : Lookup  InputValues=[-0.0400000000000091;49.96;99.96;199.96;299.96;399.96;499.96;599.96;699.96;799.96]  Table=[1;1.0375;1.075;1.15;1.2;1.25;1.3;1.35;1.4;1.4]  LookUpMeth=Interpolation-Use End Values
  Lookup_7 : Lookup  InputValues=[-100.04;-0.0400000000000091;99.96;199.96;299.96;399.96;499.96;599.96;699.96;799.96]  Table=[1;1.019;1.07;1.14;1.195;1.217;1.225;1.234;1.243;1.27]  LookUpMeth=Interpolation-Use End Values
  cpCatBrick : Outport
  cpEGBrick : Outport  Port=2
  wires:
  tBrickUs/1 -> Lookup_7/1
  Lookup_7/1 -> cpEGBrick/1
  Lookup_6/1 -> cpCatBrick/1
  tBrickDs/1 -> Lookup_6/1

== system Virtual_Exhaust_Aftertreatment_Controller_PRT/UCatCtrl/SCR_Prediction/Main/UCat Temperature Prediction/Gas and Catalyst Properties4 ==
  tBrickUs : Inport
  tBrickDs : Inport  Port=2
  Lookup_8 : Lookup  InputValues=[-0.0400000000000091;49.96;99.96;199.96;299.96;399.96;499.96;599.96;699.96;799.96]  Table=[1;1.0375;1.075;1.15;1.2;1.25;1.3;1.35;1.4;1.4]  LookUpMeth=Interpolation-Use End Values
  Lookup_9 : Lookup  InputValues=[-100.04;-0.0400000000000091;99.96;199.96;299.96;399.96;499.96;599.96;699.96;799.96]  Table=[1;1.019;1.07;1.14;1.195;1.217;1.225;1.234;1.243;1.27]  LookUpMeth=Interpolation-Use End Values
  cpCatBrick : Outport
  cpEGBrick : Outport  Port=2
  wires:
  tBrickUs/1 -> Lookup_9/1
  Lookup_9/1 -> cpEGBrick/1
  Lookup_8/1 -> cpCatBrick/1
  tBrickDs/1 -> Lookup_8/1

== system Virtual_Exhaust_Aftertreatment_Controller_PRT/UCatCtrl/Urea_Dosing_Control/Dosing Limitation/DepLimCor/ Calc facOpMode ==
  SCR_tUCatUsT : Inport
  stOpModeAct : Inport  Port=2
  Lookup_n-D_1 : Lookup_n-D  NumberOfTableDimensions=1  BreakpointsForDimension1=[158.96;159.96;179.96;199.96;219.96;229.96;239.96;249.96;299.96;319.96;339.96;359.96;379.96;399.96;499.96;599.96]  BreakpointsForDimension2=[159.96 449.96]  Table=[0;0;1;1;1;1;1;1;1;1;1;1;1;1;1;1]  ExtrapMethod=Clip  UseLastTableValue=on  RndMeth=Simplest  InputSameDT=on
  Lookup_n-D_2 : Lookup_n-D  NumberOfTableDimensions=1  BreakpointsForDimension1=[158.96;159.96;179.96;199.96;219.96;229.96;239.96;249.96;299.96;319.96;339.96;359.96;379.96;399.96;499.96;599.96]  BreakpointsForDimension2=[159.96 449.96]  Table=[0;0;1;1;1;1;1;1;1;1;1;1;1;1;1;1]  ExtrapMethod=Clip  UseLastTableValue=on  RndMeth=Simplest  InputSameDT=on
  Lookup_n-D_3 : Lookup_n-D  NumberOfTableDimensions=1  BreakpointsForDimension1=[158.96;169.96;179.96;184.96;189.96;194.96;199.96;204.96;209.96;214.96;219.96;224.96;239.96;249.96;274.96;299.96]  BreakpointsForDimension2=[159.96 449.96]  Table=[0;0;1;1;1;1;1;1;1;1;1;1;1;1;1;1]  ExtrapMethod=Clip  UseLastTableValue=on  RndMeth=Simplest  InputSameDT=on
  Lookup_n-D_4 : Lookup_n-D  NumberOfTableDimensions=1  BreakpointsForDimension1=[158.96;169.96;179.96;184.96;189.96;194.96;199.96;204.96;209.96;214.96;219.96;224.96;239.96;249.96;274.96;299.96]  BreakpointsForDimension2=[159.96 449.96]  Table=[0;0;0;0;1;1;1;1;1;1;1;1;1;1;1;1]  ExtrapMethod=Clip  UseLastTableValue=on  RndMeth=Simplest  InputSameDT=on
  MultiSw1 : MultiPortSwitch  DataPortOrder=Zero-based contiguous  Inputs=6  zeroidx=on
  DepLimCor_facOpMode : Outport
  wires:
  SCR_tUCatUsT/1 -> Lookup_n-D_2/1, Lookup_n-D_4/1, Lookup_n-D_3/1, Lookup_n-D_1/1
  stOpModeAct/1 -> MultiSw1/1
  Lookup_n-D_1/1 -> MultiSw1/3, MultiSw1/7, MultiSw1/2  "DepLimCor_facOpMode0_mp"
  Lookup_n-D_2/1 -> MultiSw1/4  "DepLimCor_facOpMode2_mp"
  Lookup_n-D_3/1 -> MultiSw1/5  "DepLimCor_facOpMode3_mp"
  Lookup_n-D_4/1 -> MultiSw1/6  "DepLimCor_facOpMode4_mp"
  MultiSw1/1 -> DepLimCor_facOpMode/1

== system Virtual_Exhaust_Aftertreatment_Controller_PRT/UCatCtrl/Urea_Dosing_Control/Dosing Limitation/DepLimCor/ Calc facOpMode_OriginalVersion ==
  SCR_tUCatUsT : Inport
  CoEOM_stOpModeAct : Inport  Port=2
  DepLimCor_facOpMode0_CUR : Lookup_n-D  NumberOfTableDimensions=1  BreakpointsForDimension1=CAL.TABLE.DepLimCor_facOpMode0_CUR.X  BreakpointsForDimension2=CAL.TABLE.SCRLdG_dmMinCor_M.X  Table=CAL.TABLE.DepLimCor_facOpMode0_CUR.Y  ExtrapMethod=Clip  UseLastTableValue=on  RndMeth=Simplest  InputSameDT=on
  DepLimCor_facOpMode2_CUR : Lookup_n-D  NumberOfTableDimensions=1  BreakpointsForDimension1=CAL.TABLE.DepLimCor_facOpMode2_CUR.X  BreakpointsForDimension2=CAL.TABLE.SCRLdG_dmMinCor_M.X  Table=CAL.TABLE.DepLimCor_facOpMode2_CUR.Y  ExtrapMethod=Clip  UseLastTableValue=on  RndMeth=Simplest  InputSameDT=on
  DepLimCor_facOpMode3_CUR : Lookup_n-D  NumberOfTableDimensions=1  BreakpointsForDimension1=CAL.TABLE.DepLimCor_facOpMode3_CUR.X  BreakpointsForDimension2=CAL.TABLE.SCRLdG_dmMinCor_M.X  Table=CAL.TABLE.DepLimCor_facOpMode3_CUR.Y  ExtrapMethod=Clip  UseLastTableValue=on  RndMeth=Simplest  InputSameDT=on
  DepLimCor_facOpMode4_CUR : Lookup_n-D  NumberOfTableDimensions=1  BreakpointsForDimension1=CAL.TABLE.DepLimCor_facOpMode4_CUR.X  BreakpointsForDimension2=CAL.TABLE.SCRLdG_dmMinCor_M.X  Table=CAL.TABLE.DepLimCor_facOpMode4_CUR.Y  ExtrapMethod=Clip  UseLastTableValue=on  RndMeth=Simplest  InputSameDT=on
  DepLimCor_facOpModeDfl_C : Constant  Value=CAL.SCALAR.DepLimCor_facOpModeDfl_C.value
  DepLimCor_idxOpMode0_C : Constant  Value=CAL.SCALAR.DepLimCor_idxOpMode0_C.value
  DepLimCor_idxOpMode2_C : Constant  Value=CAL.SCALAR.DepLimCor_idxOpMode2_C.value
  DepLimCor_idxOpMode3_C : Constant  Value=CAL.SCALAR.DepLimCor_idxOpMode3_C.value
  DepLimCor_idxOpMode4_C : Constant  Value=CAL.SCALAR.DepLimCor_idxOpMode4_C.value
  MultiportSwitch{,1..3} (4 alike) : MultiPortSwitch  DataPortOrder=Zero-based contiguous  Inputs=2
  Subsystem : Subsystem
  Subsystem1 : Subsystem
  Subsystem2 : Subsystem
  Subsystem3 : Subsystem
  T3LimCL_EOMSelection : Subsystem  Commented=on
  DepLimCor_facOpMode : Outport
  wires:
  SCR_tUCatUsT/1 -> DepLimCor_facOpMode0_CUR/1, DepLimCor_facOpMode2_CUR/1, DepLimCor_facOpMode4_CUR/1, DepLimCor_facOpMode3_CUR/1
  CoEOM_stOpModeAct/1 -> Subsystem1/1(stOpModeMsk), Subsystem3/1(stOpModeMsk), Subsystem2/1(stOpModeMsk), Subsystem/1(stOpModeMsk)
  DepLimCor_idxOpMode0_C/1 -> Subsystem/2(stOpMode)
  DepLimCor_idxOpMode2_C/1 -> Subsystem1/2(stOpMode)
  DepLimCor_idxOpMode3_C/1 -> Subsystem2/2(stOpMode)
  DepLimCor_idxOpMode4_C/1 -> Subsystem3/2(stOpMode)
  DepLimCor_facOpModeDfl_C/1 -> MultiportSwitch/2
  Subsystem3/1(Out) -> MultiportSwitch/1
  DepLimCor_facOpMode4_CUR/1 -> MultiportSwitch/3  "DepLimCor_facOpMode4_mp"
  MultiportSwitch/1 -> MultiportSwitch1/2
  Subsystem2/1(Out) -> MultiportSwitch1/1
  DepLimCor_facOpMode3_CUR/1 -> MultiportSwitch1/3  "DepLimCor_facOpMode3_mp"
  Subsystem1/1(Out) -> MultiportSwitch2/1
  DepLimCor_facOpMode2_CUR/1 -> MultiportSwitch2/3  "DepLimCor_facOpMode2_mp"
  MultiportSwitch1/1 -> MultiportSwitch2/2
  Subsystem/1(Out) -> MultiportSwitch3/1
  DepLimCor_facOpMode0_CUR/1 -> MultiportSwitch3/3  "DepLimCor_facOpMode0_mp"
  MultiportSwitch2/1 -> MultiportSwitch3/2
  MultiportSwitch3/1 -> DepLimCor_facOpMode/1

== system Virtual_Exhaust_Aftertreatment_Controller_PRT/UCatCtrl/Urea_Dosing_Control/Dosing Limitation/DepLimCor/PT1 ==
  X : Inport
  K : Inport  Port=2
  TeQ : Inport  Port=3
  Add1 : Sum  Inputs=+-
  Add2 : Sum
  Constant_2 : Constant  SampleTime=-1
  Delay1 : Delay  DelayLength=1  InitialCondition=0
  Divide1 : Product  Inputs=**
  Divide2 : Product  Inputs=***
  Y : Outport
  wires:
  Constant_2/1 -> Add1/1
  TeQ/1 -> Add1/2, Divide1/1
  Add2/1 -> Y/1, Delay1/1
  Delay1/1 -> Divide1/2
  Divide1/1 -> Add2/2
  K/1 -> Divide2/2
  X/1 -> Divide2/1
  Add1/1 -> Divide2/3
  Divide2/1 -> Add2/1

== system Virtual_Exhaust_Aftertreatment_Controller_PRT/UCatCtrl/Urea_Dosing_Control/Dosing Limitation/DepLimCor/TeQ ==
  T : Inport
  dt : Inport  Port=2
  Constant_2 : Constant  Value=-1  SampleTime=-1
  Divide2 : Product  Inputs=***
  Math Function : Math  SaturateOnIntegerOverflow=on
  TeQ : Outport
  wires:
  Constant_2/1 -> Divide2/1
  T/1 -> Divide2/2
  dt/1 -> Divide2/3
  Divide2/1 -> Math Function/1
  Math Function/1 -> TeQ/1

== system Virtual_Exhaust_Aftertreatment_Controller_PRT/UCatCtrl/Urea_Dosing_Control/Dosing Limitation/GOTO_DepLimCor_facNH3MaxCor/GainXX ==
  In : Inport
  Out : Outport
  wires:
  In/1 -> Out/1

== system Virtual_Exhaust_Aftertreatment_Controller_PRT/UCatCtrl/Urea_Dosing_Control/Dosing Limitation/GOTO_SCRLdG_dmNH3Max/GainXX ==
  In : Inport
  Out : Outport
  wires:
  In/1 -> Out/1

== system Virtual_Exhaust_Aftertreatment_Controller_PRT/UCatCtrl/Urea_Dosing_Control/EvpMod/EvpMod_UCatUsTEst/PT1 ==
  X : Inport
  K : Inport  Port=2
  TeQ : Inport  Port=3
  Reset : Inport  Port=4
  XReset : Inport  Port=5
  YReset : Inport  Port=6
  Add1 : Sum  Inputs=+-
  Add2 : Sum
  Constant_2 : Constant  SampleTime=-1
  Delay1 : Delay  DelayLength=1  InitialCondition=0
  Divide1 : Product  Inputs=**
  Divide2 : Product  Inputs=***
  Multiport Switch1 : MultiPortSwitch  DataPortOrder=Zero-based contiguous  Inputs=2
  Multiport Switch2 : MultiPortSwitch  DataPortOrder=Zero-based contiguous  Inputs=2
  Y : Outport
  wires:
  Constant_2/1 -> Add1/1
  TeQ/1 -> Add1/2, Divide1/1
  Add2/1 -> Y/1, Delay1/1
  Delay1/1 -> Multiport Switch1/2
  Divide1/1 -> Add2/2
  K/1 -> Divide2/2
  X/1 -> Multiport Switch2/2
  Add1/1 -> Divide2/3
  Divide2/1 -> Add2/1
  Reset/1 -> Multiport Switch2/1, Multiport Switch1/1
  XReset/1 -> Multiport Switch2/3
  YReset/1 -> Multiport Switch1/3
  Multiport Switch1/1 -> Divide1/2
  Multiport Switch2/1 -> Divide2/1

== system Virtual_Exhaust_Aftertreatment_Controller_PRT/UCatCtrl/Urea_Dosing_Control/EvpMod/EvpMod_UCatUsTEst/Saturation Dynamic1 ==
  up : Inport
  u : Inport  Port=2
  lo : Inport  Port=3
  Data Type Duplicate : DataTypeDuplicate  DisableCoverage=on
  Data Type Propagation : S-Function  FunctionName=sfix_dtprop  Parameters=14,PropDataTypeMode,(getdatatypespecs(PropDataType,PropScaling,DblOver,0, 0, PropDataTypeMode, PropScalingMode)),IfRefDouble,IfRefSingle,IsSigned,NumBitsBase,NumBitsMult,NumBitsAdd,(sort(reshape(round(NumBitsAllowFinal), prod(size(NumBitsAllowFinal)),1))),PropScalingMode,ValuesUsedBestPrec,SlopeBase,SlopeMult,SlopeAdd,BiasBase,BiasMult,BiasAdd,DblOver  SFunctionDeploymentMode=off  EnableBusSupport=off  mask(Data Type Propagation){PropDataTypeMode=Inherit via propagation rule, PropDataType=fixdt(1, 16), IfRefDouble=double, IfRefSingle=single, IsSigned=IsSigned1, NumBitsBase=NumBits1, NumBitsMult=1, NumBitsAdd=0, NumBitsAllowFinal=1:128, PropScalingMode=Inherit via propagation rule, PropScaling=2^-10, ValuesUsedBestPrec=[5 -7], SlopeBase=Slope1, SlopeMult=1, SlopeAdd=0, BiasBase=Bias1, BiasMult=1, BiasAdd=0}
      mask prompts: PropDataTypeMode "Simulink:masks:x1PropagatedDataType_MP"; PropDataType "Simulink:masks:x11PropagatedDataTypeegFixdt116Fixdtsingle_MP"; IfRefDouble "Simulink:masks:x11IfAnyReferenceInputIsDoubleOutputIs_MP"; IfRefSingle "Simulink:masks:x12IfAnyReferenceInputIsSingleOutputIs_MP"; IsSigned "Simulink:masks:x13IsSigned_MP"; NumBitsBase "Simulink:masks:x141NumberofBitsBase_MP"; NumBitsMult "Simulink:masks:x142NumberofBitsMultiplicativeAdjustment_MP"; NumBitsAdd "Simulink:masks:x143NumberofBitsAdditiveAdjustment_MP"; NumBitsAllowFinal "Simulink:masks:x144NumberofBitsAllowableFinalValues_MP"; PropScalingMode "Simulink:masks:x2PropagatedScaling_MP"; PropScaling "Simulink:masks:x21PropagatedScalingSlopeEg29OrSlopeBiasEg1253_MP"; ValuesUsedBestPrec "Simulink:masks:x21ValuesUsedToDetermineBestPrecisionScaling_MP"; SlopeBase "Simulink:masks:x211SlopeBase_MP"; SlopeMult "Simulink:masks:x212SlopeMultiplicativeAdjustment_MP"; SlopeAdd "Simulink:masks:x213SlopeAdditiveAdjustment_MP"; BiasBase "Simulink:masks:x221BiasBase_MP"; BiasMult "Simulink:masks:x222BiasMultiplicativeAdjustment_MP"; BiasAdd "Simulink:masks:x223BiasAdditiveAdjustment_MP"
      mask help: Simulink:masks:DataTypePropagation_MD
      mask init:
      | DblOver = 0;
      mask TypeOptions PropDataTypeMode: Simulink:masks:SpecifyViaDialog | Simulink:masks:InheritViaPropagationRule
      mask Callback PropDataTypeMode: fixptdialog(gcbh)
      mask Callback PropDataType: fixptdialog(gcbh)
      mask TypeOptions IfRefDouble: Simulink:masks:double | Simulink:masks:single
      mask TypeOptions IfRefSingle: Simulink:masks:double | Simulink:masks:single
      mask TypeOptions IsSigned: Simulink:masks:IsSigned1 | Simulink:masks:IsSigned2 | Simulink:masks:IsSigned1OrIsSigned2 | Simulink:masks:TRUE | Simulink:masks:FALSE
      mask TypeOptions NumBitsBase: NumBits1 | NumBits2 | max([NumBits1 NumBits2]) | min([NumBits1 NumBits2]) | NumBits1+NumBits2
      mask TypeOptions PropScalingMode: Simulink:masks:SpecifyViaDialog | Simulink:masks:InheritViaPropagationRule | Simulink:masks:ObtainViaBestPrecision
      mask Callback PropScalingMode: fixptdialog(gcbh)
      mask TypeOptions SlopeBase: Slope1 | Slope2 | max([Slope1 Slope2]) | min([Slope1 Slope2]) | Slope1*Slope2 | Slope1/Slope2 | PosRange1 | PosRange2 | max([PosRange1 PosRange2]) | min([PosRange1 PosRange2]) | PosRange1*PosRange2 | PosRange1/PosRange2
      mask TypeOptions BiasBase: Bias1 | Bias2 | max([Bias1 Bias2]) | min([Bias1 Bias2]) | Bias1*Bias2 | Bias1/Bias2 | Bias1+Bias2 | Bias1-Bias2
      mask Display:
      | port_label('Input',1,'Ref1');
      | port_label('Input',2,'Ref2');
      | port_label('Input',3,'Prop');
  LowerRelop1 : RelationalOperator  DisableCoverage=on  Operator=>  OutDataTypeStr=boolean  RndMeth=Nearest
  Switch : Switch  Criteria=u2 ~= 0  OutDataTypeStr=Inherit: Inherit via back propagation  ZeroCross=off
  Switch2 : Switch  Criteria=u2 ~= 0  OutMin=OutMin  OutMax=OutMax  OutDataTypeStr=Inherit: Inherit via back propagation  ZeroCross=off
  UpperRelop : RelationalOperator  DisableCoverage=on  Operator=<  OutDataTypeStr=boolean  RndMeth=Nearest
  y : Outport  OutMin=OutMin  OutMax=OutMax
  wires:
  up/1 -> Switch2/1, LowerRelop1/2
  u/1 -> Data Type Propagation/2, Data Type Propagation/1, LowerRelop1/1, Switch/3, UpperRelop/1
  lo/1 -> Switch/1, UpperRelop/2
  Switch/1 -> Data Type Duplicate/2, Switch2/3, Data Type Propagation/3
  Switch2/1 -> Data Type Duplicate/1, y/1
  LowerRelop1/1 -> Switch2/2
  UpperRelop/1 -> Switch/2

== system Virtual_Exhaust_Aftertreatment_Controller_PRT/UCatCtrl/Urea_Dosing_Control/EvpMod/EvpMod_UCatUsTEst/TeQ ==
  T : Inport
  dt : Inport  Port=2
  Constant_2 : Constant  Value=-1  SampleTime=-1
  Divide2 : Product  Inputs=***
  Math Function : Math  SaturateOnIntegerOverflow=on
  TeQ : Outport
  wires:
  Constant_2/1 -> Divide2/1
  T/1 -> Divide2/2
  dt/1 -> Divide2/3
  Divide2/1 -> Math Function/1
  Math Function/1 -> TeQ/1

== system Virtual_Exhaust_Aftertreatment_Controller_PRT/UCatCtrl/Urea_Dosing_Control/Feedback Control/GOTO_ATS_facNOxCtl/GainXX ==
  In : Inport
  Out : Outport
  wires:
  In/1 -> Out/1

== system Virtual_Exhaust_Aftertreatment_Controller_PRT/UCatCtrl/Urea_Dosing_Control/Feedback Control/PIDctrl/SAT1 ==
  up : Inport
  u : Inport  Port=2
  lo : Inport  Port=3
  Data Type Duplicate : DataTypeDuplicate  DisableCoverage=on
  Data Type Propagation : S-Function  FunctionName=sfix_dtprop  Parameters=14,PropDataTypeMode,(getdatatypespecs(PropDataType,PropScaling,DblOver,0, 0, PropDataTypeMode, PropScalingMode)),IfRefDouble,IfRefSingle,IsSigned,NumBitsBase,NumBitsMult,NumBitsAdd,(sort(reshape(round(NumBitsAllowFinal), prod(size(NumBitsAllowFinal)),1))),PropScalingMode,ValuesUsedBestPrec,SlopeBase,SlopeMult,SlopeAdd,BiasBase,BiasMult,BiasAdd,DblOver  SFunctionDeploymentMode=off  EnableBusSupport=off  mask(Data Type Propagation){PropDataTypeMode=Inherit via propagation rule, PropDataType=fixdt(1, 16), IfRefDouble=double, IfRefSingle=single, IsSigned=IsSigned1, NumBitsBase=NumBits1, NumBitsMult=1, NumBitsAdd=0, NumBitsAllowFinal=1:128, PropScalingMode=Inherit via propagation rule, PropScaling=2^-10, ValuesUsedBestPrec=[5 -7], SlopeBase=Slope1, SlopeMult=1, SlopeAdd=0, BiasBase=Bias1, BiasMult=1, BiasAdd=0}
      mask prompts: PropDataTypeMode "Simulink:masks:x1PropagatedDataType_MP"; PropDataType "Simulink:masks:x11PropagatedDataTypeegFixdt116Fixdtsingle_MP"; IfRefDouble "Simulink:masks:x11IfAnyReferenceInputIsDoubleOutputIs_MP"; IfRefSingle "Simulink:masks:x12IfAnyReferenceInputIsSingleOutputIs_MP"; IsSigned "Simulink:masks:x13IsSigned_MP"; NumBitsBase "Simulink:masks:x141NumberofBitsBase_MP"; NumBitsMult "Simulink:masks:x142NumberofBitsMultiplicativeAdjustment_MP"; NumBitsAdd "Simulink:masks:x143NumberofBitsAdditiveAdjustment_MP"; NumBitsAllowFinal "Simulink:masks:x144NumberofBitsAllowableFinalValues_MP"; PropScalingMode "Simulink:masks:x2PropagatedScaling_MP"; PropScaling "Simulink:masks:x21PropagatedScalingSlopeEg29OrSlopeBiasEg1253_MP"; ValuesUsedBestPrec "Simulink:masks:x21ValuesUsedToDetermineBestPrecisionScaling_MP"; SlopeBase "Simulink:masks:x211SlopeBase_MP"; SlopeMult "Simulink:masks:x212SlopeMultiplicativeAdjustment_MP"; SlopeAdd "Simulink:masks:x213SlopeAdditiveAdjustment_MP"; BiasBase "Simulink:masks:x221BiasBase_MP"; BiasMult "Simulink:masks:x222BiasMultiplicativeAdjustment_MP"; BiasAdd "Simulink:masks:x223BiasAdditiveAdjustment_MP"
      mask help: Simulink:masks:DataTypePropagation_MD
      mask init:
      | DblOver = 0;
      mask TypeOptions PropDataTypeMode: Simulink:masks:SpecifyViaDialog | Simulink:masks:InheritViaPropagationRule
      mask Callback PropDataTypeMode: fixptdialog(gcbh)
      mask Callback PropDataType: fixptdialog(gcbh)
      mask TypeOptions IfRefDouble: Simulink:masks:double | Simulink:masks:single
      mask TypeOptions IfRefSingle: Simulink:masks:double | Simulink:masks:single
      mask TypeOptions IsSigned: Simulink:masks:IsSigned1 | Simulink:masks:IsSigned2 | Simulink:masks:IsSigned1OrIsSigned2 | Simulink:masks:TRUE | Simulink:masks:FALSE
      mask TypeOptions NumBitsBase: NumBits1 | NumBits2 | max([NumBits1 NumBits2]) | min([NumBits1 NumBits2]) | NumBits1+NumBits2
      mask TypeOptions PropScalingMode: Simulink:masks:SpecifyViaDialog | Simulink:masks:InheritViaPropagationRule | Simulink:masks:ObtainViaBestPrecision
      mask Callback PropScalingMode: fixptdialog(gcbh)
      mask TypeOptions SlopeBase: Slope1 | Slope2 | max([Slope1 Slope2]) | min([Slope1 Slope2]) | Slope1*Slope2 | Slope1/Slope2 | PosRange1 | PosRange2 | max([PosRange1 PosRange2]) | min([PosRange1 PosRange2]) | PosRange1*PosRange2 | PosRange1/PosRange2
      mask TypeOptions BiasBase: Bias1 | Bias2 | max([Bias1 Bias2]) | min([Bias1 Bias2]) | Bias1*Bias2 | Bias1/Bias2 | Bias1+Bias2 | Bias1-Bias2
      mask Display:
      | port_label('Input',1,'Ref1');
      | port_label('Input',2,'Ref2');
      | port_label('Input',3,'Prop');
  LowerRelop1 : RelationalOperator  DisableCoverage=on  Operator=>  OutDataTypeStr=boolean  RndMeth=Nearest
  Switch : Switch  Criteria=u2 ~= 0  OutDataTypeStr=Inherit: Inherit via back propagation  ZeroCross=off
  Switch2 : Switch  Criteria=u2 ~= 0  OutMin=OutMin  OutMax=OutMax  OutDataTypeStr=Inherit: Inherit via back propagation  ZeroCross=off
  UpperRelop : RelationalOperator  DisableCoverage=on  Operator=<  OutDataTypeStr=boolean  RndMeth=Nearest
  y : Outport  OutMin=OutMin  OutMax=OutMax
  wires:
  up/1 -> Switch2/1, LowerRelop1/2
  u/1 -> Data Type Propagation/2, Data Type Propagation/1, LowerRelop1/1, Switch/3, UpperRelop/1
  lo/1 -> Switch/1, UpperRelop/2
  Switch/1 -> Data Type Duplicate/2, Switch2/3, Data Type Propagation/3
  Switch2/1 -> Data Type Duplicate/1, y/1
  LowerRelop1/1 -> Switch2/2
  UpperRelop/1 -> Switch/2
